simulink model "minimum_omega_verify"  (R2019a)
settings: Solver=VariableStepAuto  StartTime=0.0  StopTime=40  RelTol=1e-3
model workspace: external: MAT-File /home/owen/Desktop/play_ground/src/system_identification_car/scripts/all_current_space_2.mat (data not in the file)
values from neighbouring files (symbols this model uses):
  Ap = [-2.58333333333  -0.957777777778; 6.08  -3.33653333333]    [all_current_space_0.mat]    (also in all_current_space_2.mat = [-7.75  -0.805; 3.12  -3.2496])
  Bp = [0.0844594594595 0.972972972973]    [all_current_space_0.mat]    (also in all_current_space_2.mat = [3.75 8.4])
  Cp = [0 1]    [all_current_space_0.mat]    (also in all_current_space_2.mat)
  Dp = 0    [all_current_space_0.mat]    (also in all_current_space_2.mat)
  KA = [0.99914515393  0.0277525115347  -0.00446849202581; -0.0277525115347  0.909546034947  0.146936049528; -0.00446849202582  -0.146936049528  0.724603883327]    [all_current_space_0.mat]    (also in all_current_space_2.mat; miu_controller.m = S.KA)
  KB = [0.00425809278186 0.0404673050461 0.0270400906943]    [all_current_space_0.mat]    (also in all_current_space_2.mat; miu_controller.m = S.KB)
  KC = [-0.0950993137051 0.986999497443 -0.879042893709]    [all_current_space_0.mat]    (also in all_current_space_2.mat; miu_controller.m = S.KC)
  KD = 0    [all_current_space_0.mat]    (also in all_current_space_2.mat; miu_controller.m = S.KD)
  KmiuA = [0.989660921573 -0.000315409143075 0.0254935474923 0.00043632189968 -0.00752351352824 -0.0347538431471 0.000315401458872 0.999999949915 5.76768498032e-06 7.65202861768e-08 -1.13784830619e-06 -6.39862169315e-06 ... (36 elements, 6x6)]    [all_current_space_0.mat]    (also in all_current_space_2.mat)
  KmiuB = [0.0187086974307 -2.61873058559e-06 -0.0374568228087 -0.000324531690516 0.0070447824654 0.0279422288483]    [all_current_space_0.mat]    (also in all_current_space_2.mat)
  KmiuC = [0.463975019958 -7.60254568744e-06 -0.913589215231 0.00986831133105 0.10255470576 -0.94070661772]    [all_current_space_0.mat]    (also in all_current_space_2.mat)
  KmiuD = -5.42610429938e-05    [all_current_space_0.mat]    (also in all_current_space_2.mat)
  Ts = 0.04    [all_current_space_0.mat]    (also in all_current_space_2.mat; limited_dynamic_0.m; limited_dynamic_1_main.m; main_matlab_script4.m)
libraries: simulink x2
settings Model: Creator=root  LastModifiedBy=owen
settings DataIOCC: ReturnWorkspaceOutputs=off
settings DebuggingCC: PregeneratedLibrarySubsystemCodeDiagnostic=none  ArithmeticOperatorsInVariantConditions=warning
settings SFSimCC: SimUseLocalCustomCode=off
settings RTWCC: RTWUseLocalCustomCode=off

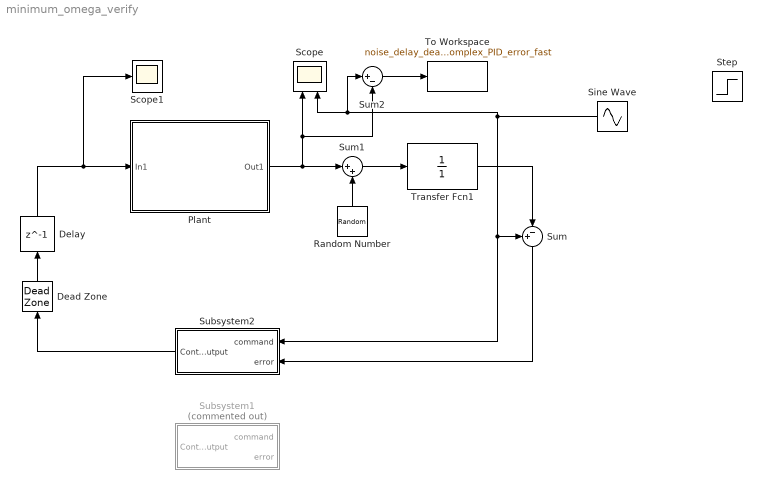
== system minimum_omega_verify ==
  Dead Zone : DeadZone  LowerValue=-0.005  UpperValue=0.005  SaturateOnIntegerOverflow=on
  Delay : Delay  DelayLength=1  SampleTime=Ts
  "Plant " : Subsystem
  Random Number : RandomNumber  Variance=0.0005  Seed=12  SampleTime=Ts
  Scope : Scope  NumInputPorts=2
  Scope1 : Scope
  Sine Wave : Sin  Amplitude=0.2  Frequency=2 * pi * 10 / 100  Phase=1  SampleTime=0
  Step : Step  Time=0  After=0.1  SampleTime=0
  Subsystem1 : Subsystem  Commented=on
  Subsystem2 : Subsystem
  Sum : Sum  Inputs=+-|
  Sum1 : Sum  Inputs=|++
  Sum2 : Sum  Inputs=|+-
  To Workspace : ToWorkspace  VariableName=noise_delay_deadzone_complex_PID_error_fast  SaveFormat=Timeseries  SampleTime=Ts
  Transfer Fcn1 : TransferFcn  Denominator=1
  wires:
  Sine Wave/1 -> Sum2/1, Scope/2, Sum/1, Subsystem2/1(command)
  Subsystem2/1(Control output) -> Dead Zone/1
  Dead Zone/1 -> Delay/1
  Delay/1 -> "Plant "/1(In1), Scope1/1
  "Plant "/1(Out1) -> Sum1/1, Sum2/2, Scope/1
  Sum1/1 -> Transfer Fcn1/1
  Random Number/1 -> Sum1/2
  Transfer Fcn1/1 -> Sum/2
  Sum2/1 -> To Workspace/1
  Sum/1 -> Subsystem2/2("error ")

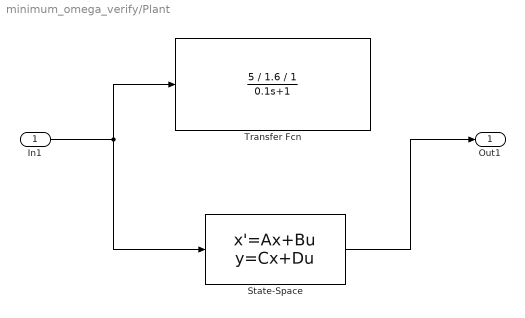
== system minimum_omega_verify/Plant  ==
  In1 : Inport
  State-Space : StateSpace  A=Ap  B=Bp  C=Cp  D=Dp  InitialCondition=0
  Transfer Fcn : TransferFcn  Numerator=5 / 1.6 / 1  Denominator=[0.1 ,1]
  Out1 : Outport
  wires:
  In1/1 -> Transfer Fcn/1, State-Space/1
  State-Space/1 -> Out1/1

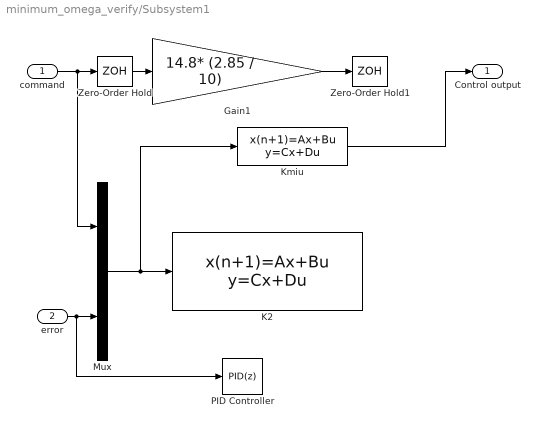
== system minimum_omega_verify/Subsystem1 ==
  command : Inport
  "error " : Inport  Port=2
  Gain1 : Gain  Gain=14.8* (2.85 / 10)
  K2 : DiscreteStateSpace  A=KA  B=KB  C=KC  D=KD  SampleTime=Ts
  Kmiu : DiscreteStateSpace  A=KmiuA  B=KmiuB  C=KmiuC  D=KmiuD  SampleTime=Ts
  Mux : Mux  Inputs=2
  PID Controller : simulink/Continuous/PID Controller  Controller=PID  TimeDomain=Discrete-time  SampleTime=Ts  IntegratorMethod=Forward Euler  FilterMethod=Forward Euler  Form=Parallel  UseFilter=off  ControllerParametersSource=internal  P=1  I=11.6  D=0.02  N=100  InitialConditionSource=internal  InitialConditionForIntegrator=0  InitialConditionForFilter=0  ExternalReset=none  LimitOutput=off  UpperSaturationLimit=inf  LowerSaturationLimit=-inf  LinearizeAsGain=on  AntiWindupMode=none  Kb=1  TrackingMode=off  Kt=1  PParamMin=[]  PParamMax=[]  IParamMin=[]  IParamMax=[]  DParamMin=[]  DParamMax=[]  NParamMin=[]  NParamMax=[]  KbParamMin=[]  KbParamMax=[]  KtParamMin=[]  KtParamMax=[]  POutMin=[]  POutMax=[]  IOutMin=[]  IOutMax=[]  DOutMin=[]  DOutMax=[]  NOutMin=[]  NOutMax=[]  KbOutMin=[]  KbOutMax=[]  KtOutMin=[]  KtOutMax=[]  IntegratorOutMin=[]  IntegratorOutMax=[]  FilterOutMin=[]  FilterOutMax=[]  SumOutMin=[]  SumOutMax=[]  SumI1OutMin=[]  SumI1OutMax=[]  SumI2OutMin=[]  SumI2OutMax=[]  SumI3OutMin=[]  SumI3OutMax=[]  SumDOutMin=[]  SumDOutMax=[]  SaturationOutMin=[]  SaturationOutMax=[]  IntegratorContinuousStateAttributes=''  IntegratorStateMustResolveToSignalObject=off  IntegratorRTWStateStorageClass=Auto  FilterContinuousStateAttributes=''  FilterStateMustResolveToSignalObject=off  FilterRTWStateStorageClass=Auto  DifferentiatorICPrevScaledInput=0  DifferentiatorOutMin=[]  DifferentiatorOutMax=[]  FilterDiffOutCoefMin=[]  FilterDiffOutCoefMax=[]  SumDenOutMin=[]  SumDenOutMax=[]  SumNumOutMin=[]  SumNumOutMax=[]  ReciprocalOutMin=[]  ReciprocalOutMax=[]  DivideOutMin=[]  DivideOutMax=[]  TunerSelectOption=Transfer Function Based (PID Tuner App)
  Zero-Order Hold : ZeroOrderHold  SampleTime=Ts
  Zero-Order Hold1 : ZeroOrderHold  SampleTime=Ts
  Control output : Outport
  wires:
  command/1 -> Mux/1, Zero-Order Hold/1
  "error "/1 -> PID Controller/1, Mux/2
  Mux/1 -> Kmiu/1, K2/1
  Gain1/1 -> Zero-Order Hold1/1
  Zero-Order Hold/1 -> Gain1/1
  Kmiu/1 -> Control output/1

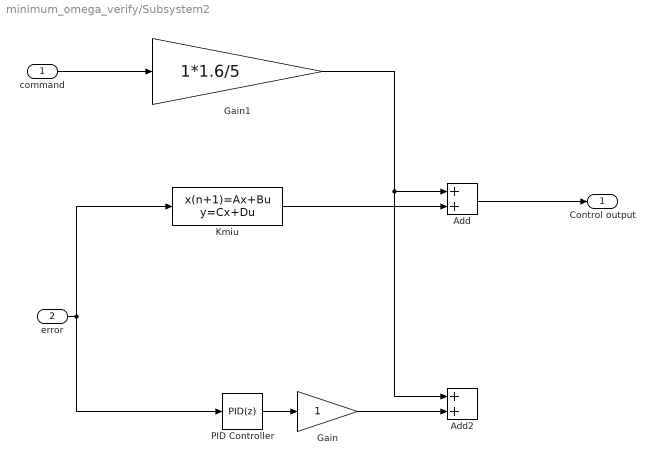
== system minimum_omega_verify/Subsystem2 ==
  command : Inport
  "error " : Inport  Port=2
  Add : Sum
  Add2 : Sum
  Gain : Gain
  Gain1 : Gain  Gain=1*1.6/5
  Kmiu : DiscreteStateSpace  A=KmiuA  B=KmiuB  C=KmiuC  D=KmiuD  SampleTime=Ts
  PID Controller : simulink/Continuous/PID Controller  Controller=PID  Form=Parallel  TimeDomain=Discrete-time  SampleTime=Ts  IntegratorMethod=Forward Euler  FilterMethod=Forward Euler  ControllerParametersSource=internal  P=0.0290918485759353  I=0.727296214398382  D=0.000290918485759352  UseFilter=off  N=100  TunerSelectOption=Transfer Function Based (PID Tuner App)  InitialConditionSource=internal  InitialConditionForIntegrator=0  InitialConditionForFilter=0  DifferentiatorICPrevScaledInput=0  ExternalReset=none  TrackingMode=off  Kt=1  LimitOutput=off  UpperSaturationLimit=inf  LowerSaturationLimit=-inf  LinearizeAsGain=on  AntiWindupMode=none  Kb=1  POutMin=[]  POutMax=[]  IOutMin=[]  IOutMax=[]  DOutMin=[]  DOutMax=[]  NOutMin=[]  NOutMax=[]  SumOutMin=[]  SumOutMax=[]  SaturationOutMin=[]  SaturationOutMax=[]  PParamMin=[]  PParamMax=[]  IParamMin=[]  IParamMax=[]  DParamMin=[]  DParamMax=[]  NParamMin=[]  NParamMax=[]  KbParamMin=[]  KbParamMax=[]  KtParamMin=[]  KtParamMax=[]  KbOutMin=[]  KbOutMax=[]  KtOutMin=[]  KtOutMax=[]  IntegratorOutMin=[]  IntegratorOutMax=[]  FilterOutMin=[]  FilterOutMax=[]  SumI1OutMin=[]  SumI1OutMax=[]  SumI2OutMin=[]  SumI2OutMax=[]  SumI3OutMin=[]  SumI3OutMax=[]  SumI4OutMin=[]  SumI4OutMax=[]  SumDOutMin=[]  SumDOutMax=[]  DifferentiatorOutMin=[]  DifferentiatorOutMax=[]  FilterDiffOutCoefMin=[]  FilterDiffOutCoefMax=[]  ReciprocalOutMin=[]  ReciprocalOutMax=[]  SumDenOutMin=[]  SumDenOutMax=[]  SumNumOutMin=[]  SumNumOutMax=[]  DivideOutMin=[]  DivideOutMax=[]  IntegratorContinuousStateAttributes=''  IntegratorStateMustResolveToSignalObject=off  IntegratorRTWStateStorageClass=Auto  FilterContinuousStateAttributes=''  FilterStateMustResolveToSignalObject=off  FilterRTWStateStorageClass=Auto  ParallelPVariant=InternalParameters  IdealPVariant=Disabled  IVariant=InternalParameters  DVariant=InternalParameters  IntegratorVariant=Discrete  SatVariant=Disabled  AWVariant=Passthrough  PCopyVariant=Disabled  TRVariant=Disabled  FdbkBlocksVariant=Forward  IdealPFdbkVariant=Disabled  SatFdbkVariant=Disabled  DerivativeFilterVariant=Differentiator  NVariant=Passthrough  NCopyVariant=Disabled_SignalSpec  FilterICVariant=InternalICsDifferentiator  IntegratorICVariant=InternalICs  ExternalResetVariant=Disabled  TRSumVariant=Passthrough  SumFdbkVariant=Disabled  SumVariant=Sum_PID
  Control output : Outport
  wires:
  "error "/1 -> Kmiu/1, PID Controller/1
  command/1 -> Gain1/1
  Kmiu/1 -> Add/2
  PID Controller/1 -> Gain/1
  Gain/1 -> Add2/2
  Gain1/1 -> Add2/1, Add/1
  Add/1 -> Control output/1
